simulink model "check_function_lookuptables"  (R2016b)
settings: Solver=VariableStepAuto  StartTime=0.0  StopTime=10.0  RelTol=1e-3
undefined symbols (not defined in the file or in its folder): look_up_table_hip, look_up_table_knee, look_up_table_x, look_up_table_y
settings Model: Creator=march  LastModifiedBy=march

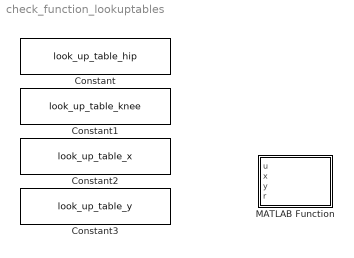
== system check_function_lookuptables ==
  Constant : Constant  Value=look_up_table_hip
  Constant1 : Constant  Value=look_up_table_knee
  Constant2 : Constant  Value=look_up_table_x
  Constant3 : Constant  Value=look_up_table_y
  MATLAB Function : MATLAB Function  TreatAsAtomicUnit=on

== matlab function check_function_lookuptables/MATLAB Function ==
  data: u input; x input; y input; r input
function fcn(u,x,y,r)

disp(u)
disp(x)
disp(u)
disp(r)
